simulink library "carnotUIBK_bus"  (R2023b)
settings: Solver=VariableStepAuto  StartTime=0.0  StopTime=10.0  RelTol=1e-3  EnableMultiTasking=on
values from neighbouring files (symbols this model uses):
  A = 7*10*2    (= 140)    [theta_ground_v1.m]    (also in xlswrite1.m = num2cell(data))
  amb_factor = 1    [DOOR.m]    (also in WALL.m; WINDOW.m = 0)
  area = obj.width * obj.height    [DOOR.m]    (also in RES.m = []; ROOM.m = 0; THERMALZONE.m = area + room(kk).area; WALL.m = area - obj.doors(jj).calc_area())
  B = A/(0.5 * P)    (= 8.23529411765)    [theta_ground_v1.m]
  boundary = BOUNDARY()    [BUILDING.m]    (also in WALL.m = '')
  building = obj    [BUILDING.m]    (also in create_building_automatic.m = building.save(); ini_building_automatic.m = building.add_variant_hvac(building.variant_hvac, hvac); load_building_automatic.m = building.save())
  C = zeros(1,length(d)+1)    [CONSTRUCTION.m]    (also in DOOR.m = [0 0 0]; WALL.m = [0 0 0]; WINDOW.m = [0 0 0])
  control = 2    [GAIN.m]    (also in GAINS.m)
  cp = str2num(value)    [CONSTRUCTION.m]
  height = 0    [DOOR.m]    (also in ROOM.m; THERMALZONE.m; WALL.m; WINDOW.m)
  p = [timevec_weather weather(:,12)]    [BOUNDARY.m]    (also in WEATHER.m = 0; init_carnotUIBK.m = cell2mat(carnotUIBKpaths(i,2)))
  rho = str2num(value)    [CONSTRUCTION.m]    (also in theta_ground_v1.m = 2000)
  type = 1    [CONSTRUCTION.m]    (also in GAINS.m = raw_moisture{ii,3}; STRUCTURE.m = 0)
  view_factor = 1    [DOOR.m]    (also in WINDOW.m = 0)
  wall = []    [ROOM.m]
  z = obj.Z    [WALL.m]    (also in theta_ground_v1.m = 0)
  zone = obj.zone(ind)    [THERMALZONE.m]
undefined symbols (not defined in the file or in its folder): const, Dd, get_building, mdot_air, mdot_CO2, mdot_H2O, mdot_VOC, pos, Qdot_C, Qdot_H, Qdot_I_electricity, Qdot_I_light, Qdot_I_person, Qdot_S, Qdot_T_ground, Qdot_T_internal, Qdot_T_neighbour, Qdot_T_opaque, Qdot_T_window, Qdot_V_infiltration, Qdot_V_mech, Qdot_V_window, Qdotc, Qdotr, r_frame, solar_ratio, solar_ratio1, solar_ratio2, Tc, Tr, Ts, Uvalue, wallsurface, window, window_height, window_heigth, window_width, windowsurface, x_CO2, x_H2O, x_VOC
libraries: $bdroot x134, carnot x87, simulink_extras x14, slpidlib x4, simulink x3
(part 10 of 12)

== system carnotUIBK_bus/wall_zone/hygrothermal model/alpha_i/alpha_i_horizontal ==
  note: (W/m^2)
  note: Convective and radiative heat transfer at the INDOOR SURFACE of a VERTICAL OUTER WALL
  note: CONVENTION:
      | Qdot > 0 and qdots < 0, if Ts > T (heat flows from wall surface to room node),
      | Qdot < 0 and qdots > 0, if Ts < T (heat flows from room node to wall surface).
  note: s: surface
      | c: convective
      | r: radiative
  note: dynamic, convective heat transfer coefficients according to: Glück B.: Wärmeübergangskoeffizienten an thermisch aktiven Bauteiloberflächen
      | und der Übergang zu Basiskennlinien für die Wärmestromdichte; gi Gesundheits-Ingenieur; 128. Jahrgang 2007, Heft 1, Seiten 1-10
  Ts : Inport
  AIB : Inport  Port=2
  Qdot sol : Inport  Port=3
  phis : Inport  Port=4
  1/wallsurface : Gain  Gain=1/wallsurface  SaturateOnIntegerOverflow=on  OutDataTypeStr=Inherit: Same as input  ParamDataTypeStr=Inherit: Same as input
  Add : Sum  Commented=on  Inputs=+-
  Bus Assignment2 : BusAssignment  AssignedSignals=Qdotc,Qdotr,mdot_H2O
  Bus Selector : BusSelector  OutputSignals=Tc,Tr,p,x_H2O
  Fcn : Fcn  Expr=1.6*(abs(u(1)-u(2)))^0.3
  Fcn1 : Fcn  Expr=(273.15+u(1))^4-(273.15+u(2))^4
  Gain2 : Gain  Commented=on  Gain=0.01
  Mux2 : Mux  Inputs=2
  Mux3 : Mux  Inputs=2
  Product : Product  InputSameDT=on  RndMeth=Zero  SaturateOnIntegerOverflow=on  OutDataTypeStr=Inherit: Same as first input
  Product1 : Product  InputSameDT=on  RndMeth=Zero  SaturateOnIntegerOverflow=on  OutDataTypeStr=Inherit: Same as first input
  Product2 : Product  Commented=on  RndMeth=Zero
  Product3 : Product  Commented=on  RndMeth=Zero
  Product4 : Product  Commented=on  InputSameDT=on  RndMeth=Zero  SaturateOnIntegerOverflow=on  OutDataTypeStr=Inherit: Same as first input
  S_initialize : $bdroot/general/S_initialize  SystemSampleTime=-1  VariantActivationTime=update diagram  AllowFlexibleInterface=on  Latency=0  AutoFrameSizeCalculation=off
  Sum : Sum  Inputs=+-  InputSameDT=on  SaturateOnIntegerOverflow=on  OutDataTypeStr=Inherit: Same as first input
  Sum2 : Sum  Inputs=+--  InputSameDT=on  SaturateOnIntegerOverflow=on  OutDataTypeStr=Inherit: Same as first input
  Switch : Switch  Commented=on  Criteria=u2 > Threshold  SaturateOnIntegerOverflow=off  InputSameDT=off
  emission_in : Gain  Gain=emission_in  SaturateOnIntegerOverflow=on  OutDataTypeStr=Inherit: Same as input  ParamDataTypeStr=Inherit: Same as input
  lewis : Gain  Commented=on  Gain=0.000000007  SaturateOnIntegerOverflow=on  OutDataTypeStr=Inherit: Same as input  ParamDataTypeStr=Inherit: Same as input
  nomassflow : Constant  Value=0
  ps_l : Fcn  Commented=on  Expr=610.0*exp(17.08*(u)/(234.2+(u)))
  ps_s_l : Fcn  Commented=on  Expr=610.0*exp(17.08*(u)/(234.2+(u)))
  sigma : Constant  Value=5.67e-8
  view_factor : Gain  Gain=view_factor  SaturateOnIntegerOverflow=on  OutDataTypeStr=Inherit: Same as input  ParamDataTypeStr=Inherit: Same as input
  wallsurface1 : Gain  Commented=on  Gain=wallsurface  SaturateOnIntegerOverflow=on  OutDataTypeStr=Inherit: Same as input  ParamDataTypeStr=Inherit: Same as input
  wallsurface2 : Gain  Gain=wallsurface  SaturateOnIntegerOverflow=on  OutDataTypeStr=Inherit: Same as input  ParamDataTypeStr=Inherit: Same as input
  wallsurface3 : Gain  Gain=wallsurface  SaturateOnIntegerOverflow=on  OutDataTypeStr=Inherit: Same as input  ParamDataTypeStr=Inherit: Same as input
  x2RelHum_UIBK : carnot/Basic/Material_Properties/x2RelHum  Commented=on
      settings: SourceProductName=Carnot
  qdots : Outport  InitialOutput=0  VectorParamsAs1DForOutWhenUnconnected=off
  "[S]" : Outport  Port=2  InitialOutput=0  VectorParamsAs1DForOutWhenUnconnected=off
  alpha_c : Outport  Port=3  InitialOutput=0  VectorParamsAs1DForOutWhenUnconnected=off
  phi_i_1/100 : Outport  Port=4  InitialOutput=0  VectorParamsAs1DForOutWhenUnconnected=off
  wires:
  wallsurface1/1 -> Switch/1
  view_factor/1 -> Product/1
  phis/1 -> Product3/1, Switch/2
  Product2/1 -> Add/2
  Product3/1 -> Add/1
  ps_s_l/1 -> Product3/2
  ps_l/1 -> Product2/2
  lewis/1 -> wallsurface1/1
  Gain2/1 -> Product2/1, phi_i_1/100/1
  Bus Selector/4 -> x2RelHum_UIBK/3  "<x_H2O>"
  Bus Selector/3 -> x2RelHum_UIBK/2  "<p>"
  x2RelHum_UIBK/1 -> Gain2/1
  Fcn1/1 -> Product/2
  Mux3/1 -> Fcn1/1
  sigma/1 -> emission_in/1
  Sum2/1 -> qdots/1
  AIB/1 -> Bus Selector/1
  Bus Selector/1 -> Sum/2, Mux2/2, x2RelHum_UIBK/1, ps_l/1  "<Tc>"
  emission_in/1 -> view_factor/1
  Product/1 -> wallsurface3/1, Sum2/3  "qdotr"
  Ts/1 -> Sum/1, ps_s_l/1, Mux3/1, Mux2/1  "Ts"
  Sum/1 -> Product1/1  "dTc"
  Bus Selector/2 -> Mux3/2  "<Tr>"
  Mux2/1 -> Fcn/1
  Product1/1 -> wallsurface2/1, Sum2/2  "qdotc"
  Fcn/1 -> alpha_c/1, Product4/1, Product1/2  "hc"
  Qdot sol/1 -> 1/wallsurface/1
  1/wallsurface/1 -> Sum2/1
  Product4/1 -> lewis/1
  Add/1 -> Product4/2
  nomassflow/1 -> Bus Assignment2/4, Switch/3
  S_initialize/1 -> Bus Assignment2/1
  wallsurface2/1 -> Bus Assignment2/2  "Qdotc"
  wallsurface3/1 -> Bus Assignment2/3  "Qdotr"
  Bus Assignment2/1 -> "[S]"/1

== system carnotUIBK_bus/wall_zone/hygrothermal model/alpha_i/alpha_i_up ==
  note: (W/m^2)
  note: Convective and radiative heat transfer at the INDOOR SURFACE of a ceiling
  note: CONVENTION:
      | Qdot > 0 and qdots < 0, if Ts > T (heat flows from wall surface to room node),
      | Qdot < 0 and qdots > 0, if Ts < T (heat flows from room node to wall surface).
  note: s: surface
      | c: convective
      | r: radiative
  note: dynamic, convective heat transfer coefficients according to: Glück B.: Wärmeübergangskoeffizienten an thermisch aktiven Bauteiloberflächen
      | und der Übergang zu Basiskennlinien für die Wärmestromdichte; gi Gesundheits-Ingenieur; 128. Jahrgang 2007, Heft 1, Seiten 1-10
  Ts : Inport
  AIB : Inport  Port=2
  Qdot sol : Inport  Port=3
  phis : Inport  Port=4
  1/wallsurface : Gain  Gain=1/wallsurface  SaturateOnIntegerOverflow=on  OutDataTypeStr=Inherit: Same as input  ParamDataTypeStr=Inherit: Same as input
  Add : Sum  Commented=on  Inputs=+-
  Bus Assignment2 : BusAssignment  AssignedSignals=Qdotc,Qdotr,mdot_H2O
  Bus Selector : BusSelector  OutputSignals=Tc,Tr,p,x_H2O
  Fcn1 : Fcn  Expr=(273.15+u(1))^4-(273.15+u(2))^4
  Gain2 : Gain  Commented=on  Gain=0.01
  Mux2 : Mux  Inputs=2
  Mux3 : Mux  Inputs=2
  Product : Product  InputSameDT=on  RndMeth=Zero  SaturateOnIntegerOverflow=on  OutDataTypeStr=Inherit: Same as first input
  Product1 : Product  InputSameDT=on  RndMeth=Zero  SaturateOnIntegerOverflow=on  OutDataTypeStr=Inherit: Same as first input
  Product2 : Product  Commented=on  RndMeth=Zero
  Product3 : Product  Commented=on  RndMeth=Zero
  Product4 : Product  Commented=on  InputSameDT=on  RndMeth=Zero  SaturateOnIntegerOverflow=on  OutDataTypeStr=Inherit: Same as first input
  S_initialize : $bdroot/general/S_initialize  SystemSampleTime=-1  VariantActivationTime=update diagram  AllowFlexibleInterface=on  Latency=0  AutoFrameSizeCalculation=off
  Sum : Sum  Inputs=+-  InputSameDT=on  SaturateOnIntegerOverflow=on  OutDataTypeStr=Inherit: Same as first input
  Sum2 : Sum  Inputs=+--  InputSameDT=on  SaturateOnIntegerOverflow=on  OutDataTypeStr=Inherit: Same as first input
  Switch : Switch  Commented=on  Criteria=u2 > Threshold  SaturateOnIntegerOverflow=off  InputSameDT=off
  Switch1 : Switch  SaturateOnIntegerOverflow=off  InputSameDT=off
  emission_in : Gain  Gain=emission_in  SaturateOnIntegerOverflow=on  OutDataTypeStr=Inherit: Same as input  ParamDataTypeStr=Inherit: Same as input
  heat flux downwards : Fcn  Expr=0.54*(abs(u(1)-u(2))^0.31)
  heat flux upwards : Fcn  Expr=2*(abs(u(1)-u(2))^0.31)
  lewis : Gain  Commented=on  Gain=0.000000007  SaturateOnIntegerOverflow=on  OutDataTypeStr=Inherit: Same as input  ParamDataTypeStr=Inherit: Same as input
  nomassflow : Constant  Value=0
  ps_l : Fcn  Commented=on  Expr=610.0*exp(17.08*(u)/(234.2+(u)))
  ps_s_l : Fcn  Commented=on  Expr=610.0*exp(17.08*(u)/(234.2+(u)))
  sigma : Constant  Value=5.67e-8
  view_factor : Gain  Gain=view_factor  SaturateOnIntegerOverflow=on  OutDataTypeStr=Inherit: Same as input  ParamDataTypeStr=Inherit: Same as input
  wallsurface1 : Gain  Commented=on  Gain=wallsurface  SaturateOnIntegerOverflow=on  OutDataTypeStr=Inherit: Same as input  ParamDataTypeStr=Inherit: Same as input
  wallsurface2 : Gain  Gain=wallsurface  SaturateOnIntegerOverflow=on  OutDataTypeStr=Inherit: Same as input  ParamDataTypeStr=Inherit: Same as input
  wallsurface3 : Gain  Gain=wallsurface  SaturateOnIntegerOverflow=on  OutDataTypeStr=Inherit: Same as input  ParamDataTypeStr=Inherit: Same as input
  x2RelHum_UIBK : carnot/Basic/Material_Properties/x2RelHum  Commented=on
      settings: SourceProductName=Carnot
  qdots : Outport  InitialOutput=0  VectorParamsAs1DForOutWhenUnconnected=off
  "[S]" : Outport  Port=2  InitialOutput=0  VectorParamsAs1DForOutWhenUnconnected=off
  alpha_c : Outport  Port=3  InitialOutput=0  VectorParamsAs1DForOutWhenUnconnected=off
  phi_i_1/100 : Outport  Port=4  InitialOutput=0  VectorParamsAs1DForOutWhenUnconnected=off
  wires:
  wallsurface1/1 -> Switch/1
  view_factor/1 -> Product/1
  phis/1 -> Product3/1, Switch/2
  Product2/1 -> Add/2
  Product3/1 -> Add/1
  ps_s_l/1 -> Product3/2
  ps_l/1 -> Product2/2
  lewis/1 -> wallsurface1/1
  Gain2/1 -> Product2/1, phi_i_1/100/1
  Bus Selector/4 -> x2RelHum_UIBK/3  "<x_H2O>"
  Bus Selector/3 -> x2RelHum_UIBK/2  "<p>"
  x2RelHum_UIBK/1 -> Gain2/1
  Fcn1/1 -> Product/2
  Mux3/1 -> Fcn1/1
  sigma/1 -> emission_in/1
  Sum2/1 -> qdots/1
  AIB/1 -> Bus Selector/1
  Bus Selector/1 -> Sum/2, Mux2/2, x2RelHum_UIBK/1, ps_l/1  "<Tc>"
  emission_in/1 -> view_factor/1
  Ts/1 -> Sum/1, ps_s_l/1, Mux3/1, Mux2/1  "Ts"
  Bus Selector/2 -> Mux3/2  "<Tr>"
  Mux2/1 -> heat flux downwards/1, heat flux upwards/1
  Switch1/1 -> Product1/2, Product4/1, alpha_c/1  "hc"
  Qdot sol/1 -> 1/wallsurface/1
  1/wallsurface/1 -> Sum2/1
  Sum/1 -> Switch1/2, Product1/1  "dTc"
  heat flux upwards/1 -> Switch1/3
  heat flux downwards/1 -> Switch1/1
  Product4/1 -> lewis/1
  Add/1 -> Product4/2
  S_initialize/1 -> Bus Assignment2/1
  Product/1 -> Sum2/3, wallsurface3/1  "qdotr"
  wallsurface3/1 -> Bus Assignment2/3  "Qdotr"
  wallsurface2/1 -> Bus Assignment2/2  "Qdotc"
  Product1/1 -> wallsurface2/1, Sum2/2  "qdotc"
  nomassflow/1 -> Bus Assignment2/4, Switch/3
  Bus Assignment2/1 -> "[S]"/1

== system carnotUIBK_bus/window/window_CARNOT/alfa_window_in/Irradiation into room ==
  note: Solar radiation into zone
  "[I_t]" : Inport
  "[tau]" : Inport  Port=2
  Demux : Demux  Outputs=3
      settings: DisplayOption=none
  Demux1 : Demux  Outputs=2
      settings: DisplayOption=none
  Product5 : Product  InputSameDT=on  SaturateOnIntegerOverflow=on  OutDataTypeStr=Inherit: Same as first input
  Product6 : Product  InputSameDT=on  SaturateOnIntegerOverflow=on  OutDataTypeStr=Inherit: Same as first input
  Sum1 : Sum  InputSameDT=on  SaturateOnIntegerOverflow=on  OutDataTypeStr=Inherit: Same as first input
  gvalue of glass : Gain  Gain=gvalue  SaturateOnIntegerOverflow=on  OutDataTypeStr=Inherit: Same as input  ParamDataTypeStr=Inherit: Same as input
  tau,dir(0) : Terminator
  qdot_sol : Outport  InitialOutput=0  VectorParamsAs1DForOutWhenUnconnected=off
  wires:
  gvalue of glass/1 -> qdot_sol/1
  Sum1/1 -> gvalue of glass/1
  "[tau]"/1 -> Demux/1
  Demux/1 -> Product5/1  "tau_dir(teta)"
  Demux/2 -> tau,dir(0)/1
  "[I_t]"/1 -> Demux1/1
  Demux1/2 -> Product6/1  "Idfu_t"
  Demux1/1 -> Product5/2  "Idir_t"
  Demux/3 -> Product6/2  "tau_dfu"
  Product6/1 -> Sum1/2
  Product5/1 -> Sum1/1

== system carnotUIBK_bus/window/window_CARNOT/alfa_window_in/transmission coefficient 1-2-3-4-layer(s) ==
  teta : Inport
  LUT_taualfa : Subsystem  mask(LOOK UP TABLE){}
      mask help:
      | This block delivers the standardized LIGHT TRANSMISSION COEFFICIENT of a window glass with 1, 2, 3 or 4 layers depending on the incidence angle. Each layer may be 3 to 8 mm thick.
      |
      | teta:    incidence angle = angle between surface normal and
      |                 incidence, degree
      | numlayer: number of layers within the window glass, [1,4].
      | tau:    transmission of glass layer stack, [0,1]
  Mux : Mux  Inputs=3
  numlayer : Constant  Value=numlayer
  perpendicular : Constant  Value=0
  tau,dfu - angle : Constant  Value=60
  "[tau]" : Outport  InitialOutput=0  VectorParamsAs1DForOutWhenUnconnected=off
  wires:
  LUT_taualfa/1(tau) -> "[tau]"/1
  numlayer/1 -> LUT_taualfa/2(numlayer)
  Mux/1 -> LUT_taualfa/1(teta)
  perpendicular/1 -> Mux/2
  tau,dfu - angle/1 -> Mux/3
  teta/1 -> Mux/1

== system carnotUIBK_bus/window/window_CARNOT/alfa_window_out/qp rad ==
  Ta : Inport
  Tw : Inport  Port=2
  Tsky : Inport  Port=3
  Sum : Sum  Inputs=-++  InputSameDT=on  SaturateOnIntegerOverflow=on  OutDataTypeStr=Inherit: Same as first input
  Ta*f : Fcn  Expr=(amb_factor)*(273.15+u[1])^4
  Tsky*f : Fcn  Expr=(1-amb_factor)*(273.15+u[1])^4
  Tw kel : Fcn  Expr=(273.15+u[1])^4
  qdot : Fcn  Expr=u(1)*emission_out*5.67e-8
  qprad : Outport  InitialOutput=0  VectorParamsAs1DForOutWhenUnconnected=off
  wires:
  Tsky/1 -> Tsky*f/1
  Ta/1 -> Ta*f/1
  qdot/1 -> qprad/1
  Sum/1 -> qdot/1
  Ta*f/1 -> Sum/3
  Tw/1 -> Tw kel/1
  Tw kel/1 -> Sum/1
  Tsky*f/1 -> Sum/2

== system carnotUIBK_bus/window/window_TF/alfa_window_in/transmission_absorption ==
  note: Assumption:
      | 1. gvalue = gvalue(0)
      | 2. gvalue(teta) / gvalue = tau(teta) / tau(0)
  note: 1. solar radiation into room (behind window glass layers)
      | 2. absorbed solar radiation flowing from inner window surface into zone
  sun_t : Inport
  WDB : Inport  Port=2
  control : Inport  Port=3
  Demux : Demux  Outputs=2
      settings: DisplayOption=none
  Demux1 : Demux  Outputs=3
      settings: DisplayOption=none
  LUT_taualfa : Subsystem  mask(LOOK UP TABLE){}
      mask help:
      | Normalized RADIATION TRANSMISSION COEFFICIENT of a window glass layer stack with 1, 2, 3 or 4 layers depending on the incidence angle.
      |
      | teta		: incidence angle = angle between surface normal and
      | 	                incidence direction, degree
      | numlayer	: number of layers within the window glass, [1,4].
      | tau		: transmission of glass layer stack, [0,1]
      |
      | NOTE: This block is defined for pane thickness between 3 and 6 mm.
  Mux : Mux  Inputs=2
  Product{1..4,7..8} (6 alike) : Product  InputSameDT=on  RndMeth=Zero  SaturateOnIntegerOverflow=on  OutDataTypeStr=Inherit: Same as first input
  Product11 : Product  Inputs=**  InputSameDT=on  RndMeth=Zero  SaturateOnIntegerOverflow=on  OutDataTypeStr=Inherit: Same as first input
  Shading : Subsystem
  Sum : Sum  Inputs=+-  InputSameDT=on  SaturateOnIntegerOverflow=on  OutDataTypeStr=Inherit: Same as first input
  Sum3 : Sum  InputSameDT=on  SaturateOnIntegerOverflow=on  OutDataTypeStr=Inherit: Same as first input
  const1 : Constant  Value=gvalue
  numlayer : Constant  Value=numpanes
  tau(0) : Gain  Gain=tauzero  SaturateOnIntegerOverflow=on  OutDataTypeStr=Inherit: Same as input  ParamDataTypeStr=Inherit: Same as input
  teta(taudfu) : Constant  Value=60
  qdot_abs : Outport  VectorParamsAs1DForOutWhenUnconnected=off
  qdot_sol : Outport  Port=2  VectorParamsAs1DForOutWhenUnconnected=off
  wires:
  control/1 -> Shading/2(control)
  WDB/1 -> Shading/1(WDB)
  Shading/3(f_g) -> Product4/2
  const1/1 -> Product4/1
  Product4/1 -> Product11/1
  Shading/4(f_tau) -> Product3/2
  Shading/2(f_dfu) -> Product1/2
  Shading/1(f_dir) -> Product2/2
  Product2/1 -> Product7/2
  Demux1/2 -> Product2/1  "Idir_t"
  Product1/1 -> Product8/2
  Demux1/3 -> Product1/1  "Idfu_t"
  Product3/1 -> qdot_sol/1, Sum/2
  tau(0)/1 -> Product3/1
  sun_t/1 -> Demux1/1
  LUT_taualfa/1(tau_norm) -> Demux/1  "Qdot_sol"
  Demux/1 -> Product7/1  "tau_norm(teta)"
  Product7/1 -> Sum3/1
  Product8/1 -> Sum3/2
  Sum3/1 -> Product11/2, tau(0)/1
  Demux/2 -> Product8/1  "tau_norm(60)"
  Product11/1 -> Sum/1  "qdot_room"
  Sum/1 -> qdot_abs/1
  Demux1/1 -> Mux/1  "teta"
  teta(taudfu)/1 -> Mux/2
  numlayer/1 -> LUT_taualfa/1(numlpanes)
  Mux/1 -> LUT_taualfa/2(teta)

== system carnotUIBK_bus/window/window_TF/alfa_window_out/qp rad ==
  Ta : Inport
  Tw : Inport  Port=2
  Tsky : Inport  Port=3
  Sum : Sum  Inputs=-++  InputSameDT=on  SaturateOnIntegerOverflow=on  OutDataTypeStr=Inherit: Same as first input
  Ta*f : Fcn  Expr=(amb_factor)*(273.15+u[1])^4
  Tsky*f : Fcn  Expr=(1-amb_factor)*(273.15+u[1])^4
  Tw kel : Fcn  Expr=(273.15+u[1])^4
  qdot : Fcn  Expr=u(1)*emission_out*5.67e-8
  qprad : Outport  InitialOutput=0  VectorParamsAs1DForOutWhenUnconnected=off
  wires:
  Tsky/1 -> Tsky*f/1
  Ta/1 -> Ta*f/1
  qdot/1 -> qprad/1
  Sum/1 -> qdot/1
  Ta*f/1 -> Sum/3
  Tw/1 -> Tw kel/1
  Tw kel/1 -> Sum/1
  Tsky*f/1 -> Sum/2

== system carnotUIBK_bus/window/window_TF_shading/alfa_window_in/transmission_absorption ==
  note: Assumption:
      | 1. gvalue = gvalue(0)
      | 2. gvalue(teta) / gvalue = tau(teta) / tau(0)
  note: 1. solar radiation into room (behind window glass layers)
      | 2. absorbed solar radiation flowing from inner window surface into zone
  sun_t : Inport
  WDB : Inport  Port=2
  control : Inport  Port=3
  Demux : Demux  Outputs=2
      settings: DisplayOption=none
  Demux1 : Demux  Outputs=3
      settings: DisplayOption=none
  LUT_taualfa : Subsystem  mask(LOOK UP TABLE){}
      mask help:
      | Normalized RADIATION TRANSMISSION COEFFICIENT of a window glass layer stack with 1, 2, 3 or 4 layers depending on the incidence angle.
      |
      | teta		: incidence angle = angle between surface normal and
      | 	                incidence direction, degree
      | numlayer	: number of layers within the window glass, [1,4].
      | tau		: transmission of glass layer stack, [0,1]
      |
      | NOTE: This block is defined for pane thickness between 3 and 6 mm.
  Mux : Mux  Inputs=2
  Product{1..4,7..8} (6 alike) : Product  InputSameDT=on  RndMeth=Zero  SaturateOnIntegerOverflow=on  OutDataTypeStr=Inherit: Same as first input
  Product11 : Product  Inputs=**  InputSameDT=on  RndMeth=Zero  SaturateOnIntegerOverflow=on  OutDataTypeStr=Inherit: Same as first input
  Shading : Subsystem
  Sum : Sum  Inputs=+-  InputSameDT=on  SaturateOnIntegerOverflow=on  OutDataTypeStr=Inherit: Same as first input
  Sum3 : Sum  InputSameDT=on  SaturateOnIntegerOverflow=on  OutDataTypeStr=Inherit: Same as first input
  const1 : Constant  Value=gvalue
  numlayer : Constant  Value=numpanes
  tau(0) : Gain  Gain=tauzero  SaturateOnIntegerOverflow=on  OutDataTypeStr=Inherit: Same as input  ParamDataTypeStr=Inherit: Same as input
  teta(taudfu) : Constant  Value=60
  qdot_abs : Outport  VectorParamsAs1DForOutWhenUnconnected=off
  qdot_sol : Outport  Port=2  VectorParamsAs1DForOutWhenUnconnected=off
  wires:
  control/1 -> Shading/2(control)
  WDB/1 -> Shading/1(WDB)
  Shading/3(f_g) -> Product4/2
  const1/1 -> Product4/1
  Product4/1 -> Product11/1
  Shading/4(f_tau) -> Product3/2
  Shading/2(f_dfu) -> Product1/2
  Shading/1(f_dir) -> Product2/2
  Product2/1 -> Product7/2
  Demux1/2 -> Product2/1  "Idir_t"
  Product1/1 -> Product8/2
  Demux1/3 -> Product1/1  "Idfu_t"
  Product3/1 -> qdot_sol/1, Sum/2
  tau(0)/1 -> Product3/1
  sun_t/1 -> Demux1/1
  LUT_taualfa/1(tau_norm) -> Demux/1  "Qdot_sol"
  Demux/1 -> Product7/1  "tau_norm(teta)"
  Product7/1 -> Sum3/1
  Product8/1 -> Sum3/2
  Sum3/1 -> Product11/2, tau(0)/1
  Demux/2 -> Product8/1  "tau_norm(60)"
  Product11/1 -> Sum/1  "qdot_room"
  Sum/1 -> qdot_abs/1
  Demux1/1 -> Mux/1  "teta"
  teta(taudfu)/1 -> Mux/2
  numlayer/1 -> LUT_taualfa/1(numlpanes)
  Mux/1 -> LUT_taualfa/2(teta)

== system carnotUIBK_bus/window/window_TF_shading/alfa_window_out/qp rad ==
  Ta : Inport
  Tw : Inport  Port=2
  Tsky : Inport  Port=3
  Sum : Sum  Inputs=-++  InputSameDT=on  SaturateOnIntegerOverflow=on  OutDataTypeStr=Inherit: Same as first input
  Ta*f : Fcn  Expr=(amb_factor)*(273.15+u[1])^4
  Tsky*f : Fcn  Expr=(1-amb_factor)*(273.15+u[1])^4
  Tw kel : Fcn  Expr=(273.15+u[1])^4
  qdot : Fcn  Expr=u(1)*emission_out*5.67e-8
  qprad : Outport  InitialOutput=0  VectorParamsAs1DForOutWhenUnconnected=off
  wires:
  Tsky/1 -> Tsky*f/1
  Ta/1 -> Ta*f/1
  qdot/1 -> qprad/1
  Sum/1 -> qdot/1
  Ta*f/1 -> Sum/3
  Tw/1 -> Tw kel/1
  Tw kel/1 -> Sum/1
  Tsky*f/1 -> Sum/2

== system carnotUIBK_bus/gain/People/W//ppl (activity)/LUT_Qdot_dry/Look-Up Table Qdot_dry ==
  Rows : Inport
  Cols : Inport  Port=2
  Look-Up Table (2-D) : Lookup2D  RowIndex=x  ColumnIndex=y  Table=t
  U : Outport  VectorParamsAs1DForOutWhenUnconnected=off
  wires:
  Look-Up Table (2-D)/1 -> U/1
  Cols/1 -> Look-Up Table (2-D)/2
  Rows/1 -> Look-Up Table (2-D)/1

== system carnotUIBK_bus/gain/People/W//ppl (activity)/LUT_Qdot_hum1/Look-Up Table Qdot_hum ==
  Rows : Inport
  Cols : Inport  Port=2
  Look-Up Table (2-D) : Lookup2D  RowIndex=x  ColumnIndex=y  Table=t
  U : Outport  VectorParamsAs1DForOutWhenUnconnected=off
  wires:
  Rows/1 -> Look-Up Table (2-D)/1
  Cols/1 -> Look-Up Table (2-D)/2
  Look-Up Table (2-D)/1 -> U/1

== system carnotUIBK_bus/gain/People/W//ppl (activity)/LUT_mdot_H2O/Look-Up Table mdot_H2O ==
  Rows : Inport
  Cols : Inport  Port=2
  Look-Up Table (2-D) : Lookup2D  RowIndex=x  ColumnIndex=y  Table=t
  U : Outport  VectorParamsAs1DForOutWhenUnconnected=off
  wires:
  Rows/1 -> Look-Up Table (2-D)/1
  Cols/1 -> Look-Up Table (2-D)/2
  Look-Up Table (2-D)/1 -> U/1

== system carnotUIBK_bus/gain/People/W//ppl (constant)/LUT_mdot_H2O/Look-Up Table mdot_H2O ==
  Rows : Inport
  Cols : Inport  Port=2
  Look-Up Table (2-D) : Lookup2D  RowIndex=x  ColumnIndex=y  Table=t
  U : Outport  VectorParamsAs1DForOutWhenUnconnected=off
  wires:
  Rows/1 -> Look-Up Table (2-D)/1
  Cols/1 -> Look-Up Table (2-D)/2
  Look-Up Table (2-D)/1 -> U/1

== system carnotUIBK_bus/infiltration/infiltration_pressure/infiltration_pressure/dP_infiltration/calculate wind_coeff ==
  wind_angle : Inport
  additional_coeff_wind : Inport  Port=2
  facade_angle : Inport  Port=3
  Cin (see ASHRAE 24.4) : Constant  Value=0.2
  Cs (see ASHRAE 24.5) : Polyval  Coefs=[0.0000005, -0.00008, -0.0074, 0.674]
  Product2 : Product
  Subtract : Sum  Inputs=-++
  Subtract1 : Sum  Inputs=+-
  const_angle : Constant  Value=180
  wind_coeff : Outport  VectorParamsAs1DForOutWhenUnconnected=off
  wires:
  wind_angle/1 -> Subtract/1
  additional_coeff_wind/1 -> Product2/2
  Product2/1 -> wind_coeff/1
  facade_angle/1 -> Subtract/3
  Subtract/1 -> Cs (see ASHRAE 24.5)/1
  const_angle/1 -> Subtract/2
  Cin (see ASHRAE 24.4)/1 -> Subtract1/2
  Subtract1/1 -> Product2/1
  Cs (see ASHRAE 24.5)/1 -> Subtract1/1

== system carnotUIBK_bus/wall_zone/R-C model/alpha_e/alpha_e_AMBIENT/qp rad ==
  Ta : Inport
  Tw : Inport  Port=2
  Tsky : Inport  Port=3
  Sum : Sum  Inputs=-++  InputSameDT=on  SaturateOnIntegerOverflow=on  OutDataTypeStr=Inherit: Same as first input
  Ta*f : Fcn  Expr=(amb_factor)*(273.15+u[1])^4
  Tsky*f : Fcn  Expr=(1-amb_factor)*(273.15+u[1])^4
  Tw kel : Fcn  Expr=(273.15+u[1])^4
  qdot : Fcn  Expr=u(1)*emission_out*5.67e-8
  qprad : Outport  InitialOutput=0  VectorParamsAs1DForOutWhenUnconnected=off
  wires:
  Tsky*f/1 -> Sum/2
  Tw kel/1 -> Sum/1
  Tw/1 -> Tw kel/1
  Ta*f/1 -> Sum/3
  Sum/1 -> qdot/1
  qdot/1 -> qprad/1
  Ta/1 -> Ta*f/1
  Tsky/1 -> Tsky*f/1

== system carnotUIBK_bus/wall_zone/R-C model/alpha_e/alpha_e_AMBIENT/wall_surfrad ==
  note: (3 = Sky model
      | Perez)
  note: Direct and diffuse
      | radiation on a
      | tilted and shaded
      | outdoor surface
  WDB : Inport
  Bus Selector : BusSelector  OutputSignals=Solar_Radiation_direct_surface,Solar_Radiation_diffuse_surface  OutputAsBus=on
  Radiation_on_Inclined_Surface : carnot/Weather/Radiation_on_Inclined_Surface  sky=Perez 1990  reflect=0.2
      settings: SourceProductName=Carnot
  Sum : Sum  Inputs=1  InputSameDT=on  SaturateOnIntegerOverflow=on  OutDataTypeStr=Inherit: Same as first input
  position : Constant  Value=pos
  Idir,t+Idfu,t : Outport  InitialOutput=0  VectorParamsAs1DForOutWhenUnconnected=off
  wires:
  Bus Selector/1 -> Sum/1
  Radiation_on_Inclined_Surface/1 -> Bus Selector/1
  Sum/1 -> Idir,t+Idfu,t/1
  WDB/1 -> Radiation_on_Inclined_Surface/1
  position/1 -> Radiation_on_Inclined_Surface/2

== system carnotUIBK_bus/wall_zone/R-C model/alpha_e/alpha_e_INTERNAL/alpha_i ==
  Ts : Inport
  AIB : Inport  Port=2
  Qdot sol : Inport  Port=3
  phis : Inport  Port=4
  alpha_i_down : Subsystem  VariantControl=V_zXXX_wXXX_hti2  mask(ALFA){}
      mask help:
      | Convective and radiative heat transfer at the INDOOR SURFACE of a VERTICAL OUTER WALL.
      |
      | [AIV] : conditions of zone node,
      | Ts : temperature of wall surface, °C,
      | qdots : specific heat flow into wall construction, W/m^2,
      | [S] : heat and air flow to zone node.
  alpha_i_horizontal : Subsystem  VariantControl=V_zXXX_wXXX_hti0  mask(ALFA){}
      mask help:
      | Convective and radiative heat transfer at the INDOOR SURFACE of a VERTICAL OUTER WALL.
      |
      | [AIV] : conditions of zone node,
      | Ts : temperature of wall surface, °C,
      | qdots : specific heat flow into wall construction, W/m^2,
      | [S] : heat and air flow to zone node.
  alpha_i_up : Subsystem  VariantControl=V_zXXX_wXXX_hti1  mask(ALFA){}
      mask help:
      | Convective and radiative heat transfer at the INDOOR SURFACE of a VERTICAL OUTER WALL.
      |
      | [AIV] : conditions of zone node,
      | Ts : temperature of wall surface, °C,
      | qdots : specific heat flow into wall construction, W/m^2,
      | [S] : heat and air flow to zone node.
  qdots : Outport  VectorParamsAs1DForOutWhenUnconnected=off
  "[S]" : Outport  Port=2  VectorParamsAs1DForOutWhenUnconnected=off
  alpha_c : Outport  Port=3  VectorParamsAs1DForOutWhenUnconnected=off
  phi_i_1/100 : Outport  Port=4  VectorParamsAs1DForOutWhenUnconnected=off

== system carnotUIBK_bus/wall_zone/R-C model/alpha_e/alpha_e_NEIGHBOUR/alpha_i ==
  Ts : Inport
  AIB : Inport  Port=2
  Qdot sol : Inport  Port=3
  phis : Inport  Port=4
  alpha_i_down : Subsystem  VariantControl=V_zXXX_wXXX_hti2  mask(ALFA){}
      mask help:
      | Convective and radiative heat transfer at the INDOOR SURFACE of a VERTICAL OUTER WALL.
      |
      | [AIV] : conditions of zone node,
      | Ts : temperature of wall surface, °C,
      | qdots : specific heat flow into wall construction, W/m^2,
      | [S] : heat and air flow to zone node.
  alpha_i_horizontal : Subsystem  VariantControl=V_zXXX_wXXX_hti0  mask(ALFA){}
      mask help:
      | Convective and radiative heat transfer at the INDOOR SURFACE of a VERTICAL OUTER WALL.
      |
      | [AIV] : conditions of zone node,
      | Ts : temperature of wall surface, °C,
      | qdots : specific heat flow into wall construction, W/m^2,
      | [S] : heat and air flow to zone node.
  alpha_i_up : Subsystem  VariantControl=V_zXXX_wXXX_hti1  mask(ALFA){}
      mask help:
      | Convective and radiative heat transfer at the INDOOR SURFACE of a VERTICAL OUTER WALL.
      |
      | [AIV] : conditions of zone node,
      | Ts : temperature of wall surface, °C,
      | qdots : specific heat flow into wall construction, W/m^2,
      | [S] : heat and air flow to zone node.
  qdots : Outport  VectorParamsAs1DForOutWhenUnconnected=off
  "[S]" : Outport  Port=2  VectorParamsAs1DForOutWhenUnconnected=off
  alpha_c : Outport  Port=3  VectorParamsAs1DForOutWhenUnconnected=off
  phi_i_1/100 : Outport  Port=4  VectorParamsAs1DForOutWhenUnconnected=off

== system carnotUIBK_bus/wall_zone/hygrothermal model/alpha_e/alpha_e_AMBIENT/qp rad ==
  Ta : Inport
  Tw : Inport  Port=2
  Tsky : Inport  Port=3
  Sum : Sum  Inputs=-++  InputSameDT=on  SaturateOnIntegerOverflow=on  OutDataTypeStr=Inherit: Same as first input
  Ta*f : Fcn  Expr=(amb_factor)*(273.15+u[1])^4
  Tsky*f : Fcn  Expr=(1-amb_factor)*(273.15+u[1])^4
  Tw kel : Fcn  Expr=(273.15+u[1])^4
  qdot : Fcn  Expr=u(1)*emission_out*5.67e-8
  qprad : Outport  InitialOutput=0  VectorParamsAs1DForOutWhenUnconnected=off
  wires:
  Tsky*f/1 -> Sum/2
  Tw kel/1 -> Sum/1
  Tw/1 -> Tw kel/1
  Ta*f/1 -> Sum/3
  Sum/1 -> qdot/1
  qdot/1 -> qprad/1
  Ta/1 -> Ta*f/1
  Tsky/1 -> Tsky*f/1

== system carnotUIBK_bus/wall_zone/hygrothermal model/alpha_e/alpha_e_AMBIENT/wall_surfrad ==
  note: (3 = Sky model
      | Perez)
  note: Direct and diffuse
      | radiation on a
      | tilted and shaded
      | outdoor surface
  WDB : Inport
  Bus Selector : BusSelector  OutputSignals=Solar_Radiation_direct_surface,Solar_Radiation_diffuse_surface  OutputAsBus=on
  Radiation_on_Inclined_Surface : carnot/Weather/Radiation_on_Inclined_Surface  sky=Perez 1990  reflect=0.2
      settings: SourceProductName=Carnot
  Sum : Sum  Inputs=1  InputSameDT=on  SaturateOnIntegerOverflow=on  OutDataTypeStr=Inherit: Same as first input
  position : Constant  Value=pos
  Idir,t+Idfu,t : Outport  InitialOutput=0  VectorParamsAs1DForOutWhenUnconnected=off
  wires:
  Bus Selector/1 -> Sum/1
  Radiation_on_Inclined_Surface/1 -> Bus Selector/1
  Sum/1 -> Idir,t+Idfu,t/1
  WDB/1 -> Radiation_on_Inclined_Surface/1
  position/1 -> Radiation_on_Inclined_Surface/2

== system carnotUIBK_bus/wall_zone/hygrothermal model/alpha_e/alpha_e_INTERNAL/alpha_i ==
  Ts : Inport
  AIB : Inport  Port=2
  Qdot sol : Inport  Port=3
  phis : Inport  Port=4
  alpha_i_down : Subsystem  VariantControl=V_zXXX_wXXX_hti2  mask(ALFA){}
      mask help:
      | Convective and radiative heat transfer at the INDOOR SURFACE of a VERTICAL OUTER WALL.
      |
      | [AIV] : conditions of zone node,
      | Ts : temperature of wall surface, °C,
      | qdots : specific heat flow into wall construction, W/m^2,
      | [S] : heat and air flow to zone node.
  alpha_i_horizontal : Subsystem  VariantControl=V_zXXX_wXXX_hti0  mask(ALFA){}
      mask help:
      | Convective and radiative heat transfer at the INDOOR SURFACE of a VERTICAL OUTER WALL.
      |
      | [AIV] : conditions of zone node,
      | Ts : temperature of wall surface, °C,
      | qdots : specific heat flow into wall construction, W/m^2,
      | [S] : heat and air flow to zone node.
  alpha_i_up : Subsystem  VariantControl=V_zXXX_wXXX_hti1  mask(ALFA){}
      mask help:
      | Convective and radiative heat transfer at the INDOOR SURFACE of a VERTICAL OUTER WALL.
      |
      | [AIV] : conditions of zone node,
      | Ts : temperature of wall surface, °C,
      | qdots : specific heat flow into wall construction, W/m^2,
      | [S] : heat and air flow to zone node.
  qdots : Outport  VectorParamsAs1DForOutWhenUnconnected=off
  "[S]" : Outport  Port=2  VectorParamsAs1DForOutWhenUnconnected=off
  alpha_c : Outport  Port=3  VectorParamsAs1DForOutWhenUnconnected=off
  phi_i_1/100 : Outport  Port=4  VectorParamsAs1DForOutWhenUnconnected=off

== system carnotUIBK_bus/wall_zone/hygrothermal model/alpha_e/alpha_e_NEIGHBOUR/alpha_i ==
  Ts : Inport
  AIB : Inport  Port=2
  Qdot sol : Inport  Port=3
  phis : Inport  Port=4
  alpha_i_down : Subsystem  VariantControl=V_zXXX_wXXX_hti2  mask(ALFA){}
      mask help:
      | Convective and radiative heat transfer at the INDOOR SURFACE of a VERTICAL OUTER WALL.
      |
      | [AIV] : conditions of zone node,
      | Ts : temperature of wall surface, °C,
      | qdots : specific heat flow into wall construction, W/m^2,
      | [S] : heat and air flow to zone node.
  alpha_i_horizontal : Subsystem  VariantControl=V_zXXX_wXXX_hti0  mask(ALFA){}
      mask help:
      | Convective and radiative heat transfer at the INDOOR SURFACE of a VERTICAL OUTER WALL.
      |
      | [AIV] : conditions of zone node,
      | Ts : temperature of wall surface, °C,
      | qdots : specific heat flow into wall construction, W/m^2,
      | [S] : heat and air flow to zone node.
  alpha_i_up : Subsystem  VariantControl=V_zXXX_wXXX_hti1  mask(ALFA){}
      mask help:
      | Convective and radiative heat transfer at the INDOOR SURFACE of a VERTICAL OUTER WALL.
      |
      | [AIV] : conditions of zone node,
      | Ts : temperature of wall surface, °C,
      | qdots : specific heat flow into wall construction, W/m^2,
      | [S] : heat and air flow to zone node.
  qdots : Outport  VectorParamsAs1DForOutWhenUnconnected=off
  "[S]" : Outport  Port=2  VectorParamsAs1DForOutWhenUnconnected=off
  alpha_c : Outport  Port=3  VectorParamsAs1DForOutWhenUnconnected=off
  phi_i_1/100 : Outport  Port=4  VectorParamsAs1DForOutWhenUnconnected=off

== system carnotUIBK_bus/window/window_CARNOT/alfa_window_in/transmission coefficient 1-2-3-4-layer(s)/LUT_taualfa ==
  note: NOTE: The TAUALFA-Lookup-table is calculated with "taualfa.m"
      | for 4 mm glass, but you can use it also for  3, 4, 6 or 8 mm glass.
      | The mistake is neglectable (see results in "taulut.m").
  note: transmission coefficient TAUALFA of a window glass with 1,2,3 or 4 layers
  note: (from: Duffie / Beckman: Solar Engineering of Thermal Processes, 1991
  teta : Inport
  numlayer : Inport  Port=2
  "TAUALFA 1-2-3-4 layers, standardized to 1.0, (4 mm float glass, no dirt absorption, 97% room absorption)" : Subsystem  mask(Lookup Table (2-D)){x=[0:10:90], y=[1:4], t=[1.0000 1.0000 1.0000 1.0000; 0.9996 0.9991 0.9987 0.9983; 0.9979 0.9961 0.9945 0.9929; 0.9937 0.9894 0.9861 0.9836; 0.9839 0.9753 0.9704 0.9680; 0.9608 0.9438 0.9365 0.9361; 0.9061 0.8679 0.8484 0.8413; 0.7755 0.6821 0.6182 0.5717; 0.4807 0.3277 0.2324 0.1688; 0 0 0 0]}
      mask prompts: x "Row:"; y "Column:"; t "Table:"
      mask help: Performs 2-D linear interpolation of input values using the specified input/output table. Extrapolation is performed outside the table boundaries.
      mask init:
      | [r,c]=size(t);
      | xt=reshape(x,prod(size(x)),1);
      | xi=xt(:,ones(1,c));
      | minx=min(x); maxx=max(x);
      | mint=min(min(t)); maxt=max(max(t));
      mask Display: plot(xi,t,[minx maxx],[mint mint],[minx minx],[mint maxt])
  tau : Outport  InitialOutput=0  VectorParamsAs1DForOutWhenUnconnected=off
  wires:
  teta/1 -> "TAUALFA 1-2-3-4 layers, standardized to 1.0, (4 mm float glass, no dirt absorption, 97% room absorption)"/1(Rows)
  numlayer/1 -> "TAUALFA 1-2-3-4 layers, standardized to 1.0, (4 mm float glass, no dirt absorption, 97% room absorption)"/2(Cols)
  "TAUALFA 1-2-3-4 layers, standardized to 1.0, (4 mm float glass, no dirt absorption, 97% room absorption)"/1(Out1) -> tau/1

== system carnotUIBK_bus/window/window_TF/alfa_window_in/transmission_absorption/LUT_taualfa ==
  note: NOTE:
      | TAUALFA-Lookup-table calculated with "taualfa.m":
      |   a) 4mm float glass (error neglectable if glass thickness is 3 or 6mm),
      |   b) no dirt absorption on glass surfaces,
      |   c) 100% room absorption,
      |   d) normalized to tau(0).
      |
      | From: Duffie / Beckman: Solar Engineering of Thermal Processes, 1991
  note: Normalized radiation transmission TAUALFA
      | of a window glass stack with 1,2,3 or 4 layers
  numlpanes : Inport
  teta : Inport  Port=2
  TAUALFA 1-2-3-4 layers : Lookup2D  RowIndex=[0:10:90]  ColumnIndex=[1:4]  Table="[1  1  1  1;.99955 .99912  .9987 .99827;.99787  .9961 .99449 .99298;.99364 .98941 .98618 .98366;.98364 .97519 .97041 .96824;.9601 .94337 .93638 .93624;.90423 .86634 .84734 .84064;.77129 .67843 .61507 .56891;.47436  .3235 .22952 .16682;0  0  0  0]"
  tau_norm : Outport  VectorParamsAs1DForOutWhenUnconnected=off
  wires:
  teta/1 -> TAUALFA 1-2-3-4 layers/1
  numlpanes/1 -> TAUALFA 1-2-3-4 layers/2
  TAUALFA 1-2-3-4 layers/1 -> tau_norm/1

== system carnotUIBK_bus/window/window_TF/alfa_window_in/transmission_absorption/Shading ==
  WDB : Inport
  control : Inport  Port=2
  Bus Selector : BusSelector  OutputSignals=Zenith_Angle
  Demux : Demux
  Mux : Mux  Inputs=2
  S-Function : S-Function  FunctionName=venetian  Parameters=bli_a, bli_b, bli_c, bli_d, bli_alpha, bli_refl, shad_type, type_glazing, tau_shad  SFunctionDeploymentMode=off  EnableBusSupport=off
  f_dir : Outport  VectorParamsAs1DForOutWhenUnconnected=off
  f_dfu : Outport  Port=2  VectorParamsAs1DForOutWhenUnconnected=off
  f_g : Outport  Port=3  VectorParamsAs1DForOutWhenUnconnected=off
  f_tau : Outport  Port=4  VectorParamsAs1DForOutWhenUnconnected=off
  wires:
  WDB/1 -> Bus Selector/1
  Bus Selector/1 -> Mux/2  "<Zenith_Angle>"
  control/1 -> Mux/1
  Mux/1 -> S-Function/1
  S-Function/1 -> Demux/1
  Demux/1 -> f_dir/1
  Demux/2 -> f_dfu/1
  Demux/3 -> f_g/1
  Demux/4 -> f_tau/1

== system carnotUIBK_bus/window/window_TF_shading/alfa_window_in/transmission_absorption/LUT_taualfa ==
  note: NOTE:
      | TAUALFA-Lookup-table calculated with "taualfa.m":
      |   a) 4mm float glass (error neglectable if glass thickness is 3 or 6mm),
      |   b) no dirt absorption on glass surfaces,
      |   c) 100% room absorption,
      |   d) normalized to tau(0).
      |
      | From: Duffie / Beckman: Solar Engineering of Thermal Processes, 1991
  note: Normalized radiation transmission TAUALFA
      | of a window glass stack with 1,2,3 or 4 layers
  numlpanes : Inport
  teta : Inport  Port=2
  TAUALFA 1-2-3-4 layers : Lookup2D  RowIndex=[0:10:90]  ColumnIndex=[1:4]  Table="[1  1  1  1;.99955 .99912  .9987 .99827;.99787  .9961 .99449 .99298;.99364 .98941 .98618 .98366;.98364 .97519 .97041 .96824;.9601 .94337 .93638 .93624;.90423 .86634 .84734 .84064;.77129 .67843 .61507 .56891;.47436  .3235 .22952 .16682;0  0  0  0]"
  tau_norm : Outport  VectorParamsAs1DForOutWhenUnconnected=off
  wires:
  teta/1 -> TAUALFA 1-2-3-4 layers/1
  numlpanes/1 -> TAUALFA 1-2-3-4 layers/2
  TAUALFA 1-2-3-4 layers/1 -> tau_norm/1

== system carnotUIBK_bus/window/window_TF_shading/alfa_window_in/transmission_absorption/Shading ==
  WDB : Inport
  control : Inport  Port=2
  Bus Selector : BusSelector  OutputSignals=Zenith_Angle
  Demux : Demux
  Mux : Mux  Inputs=2
  S-Function : S-Function  FunctionName=venetian  Parameters=bli_a, bli_b, bli_c, bli_d, bli_alpha, bli_refl, shad_type, type_glazing, tau_shad  SFunctionDeploymentMode=off  EnableBusSupport=off
  f_dir : Outport  VectorParamsAs1DForOutWhenUnconnected=off
  f_dfu : Outport  Port=2  VectorParamsAs1DForOutWhenUnconnected=off
  f_g : Outport  Port=3  VectorParamsAs1DForOutWhenUnconnected=off
  f_tau : Outport  Port=4  VectorParamsAs1DForOutWhenUnconnected=off
  wires:
  WDB/1 -> Bus Selector/1
  Bus Selector/1 -> Mux/2  "<Zenith_Angle>"
  control/1 -> Mux/1
  Mux/1 -> S-Function/1
  S-Function/1 -> Demux/1
  Demux/1 -> f_dir/1
  Demux/2 -> f_dfu/1
  Demux/3 -> f_g/1
  Demux/4 -> f_tau/1

== system carnotUIBK_bus/wall_zone/R-C model/alpha_e/alpha_e_INTERNAL/alpha_i/alpha_i_down ==
  note: (W/m^2)
  note: Convective and radiative heat transfer at the INDOOR SURFACE of a VERTICAL OUTER WALL
  note: CONVENTION:
      | Qdot > 0 and qdots < 0, if Ts > T (heat flows from wall surface to room node),
      | Qdot < 0 and qdots > 0, if Ts < T (heat flows from room node to wall surface).
  note: s: surface
      | c: convective
      | r: radiative
  note: dynamic, convective heat transfer coefficients according to: Glück B.: Wärmeübergangskoeffizienten an thermisch aktiven Bauteiloberflächen
      | und der Übergang zu Basiskennlinien für die Wärmestromdichte; gi Gesundheits-Ingenieur; 128. Jahrgang 2007, Heft 1, Seiten 1-10
  Ts : Inport
  AIB : Inport  Port=2
  Qdot sol : Inport  Port=3
  phis : Inport  Port=4
  1/wallsurface : Gain  Gain=1/wallsurface  SaturateOnIntegerOverflow=on  OutDataTypeStr=Inherit: Same as input  ParamDataTypeStr=Inherit: Same as input
  Add : Sum  Commented=on  Inputs=+-
  Bus Assignment2 : BusAssignment  AssignedSignals=Qdotc,Qdotr,Qdot_T_internal,mdot_H2O
  Bus Selector : BusSelector  OutputSignals=Tc,Tr,p,x_H2O
  Fcn1 : Fcn  Expr=(273.15+u(1))^4-(273.15+u(2))^4
  Gain2 : Gain  Commented=on  Gain=0.01
  Mux2 : Mux  Inputs=2
  Mux3 : Mux  Inputs=2
  Product : Product  InputSameDT=on  RndMeth=Zero  SaturateOnIntegerOverflow=on  OutDataTypeStr=Inherit: Same as first input
  Product1 : Product  InputSameDT=on  RndMeth=Zero  SaturateOnIntegerOverflow=on  OutDataTypeStr=Inherit: Same as first input
  Product2 : Product  Commented=on  RndMeth=Zero
  Product3 : Product  Commented=on  RndMeth=Zero
  S_initialize : $bdroot/general/S_initialize  SystemSampleTime=-1  VariantActivationTime=update diagram  AllowFlexibleInterface=on  Latency=0  AutoFrameSizeCalculation=off
  Sum : Sum  Inputs=+-  InputSameDT=on  SaturateOnIntegerOverflow=on  OutDataTypeStr=Inherit: Same as first input
  Sum2 : Sum  Inputs=+--  InputSameDT=on  SaturateOnIntegerOverflow=on  OutDataTypeStr=Inherit: Same as first input
  Switch : Switch  Commented=on  Criteria=u2 > Threshold  SaturateOnIntegerOverflow=off  InputSameDT=off
  Switch1 : Switch  SaturateOnIntegerOverflow=off  InputSameDT=off
  Wallsurf : Gain  Gain=wallsurface  SaturateOnIntegerOverflow=on  OutDataTypeStr=Inherit: Same as input  ParamDataTypeStr=Inherit: Same as input
  emission_in : Gain  Gain=emission_in  SaturateOnIntegerOverflow=on  OutDataTypeStr=Inherit: Same as input  ParamDataTypeStr=Inherit: Same as input
  heat flux downwards : Fcn  Expr=0.54*(abs(u(1)-u(2))^0.31)
  heat flux upwards : Fcn  Expr=2*(abs(u(1)-u(2))^0.31)
  lewis : Gain  Commented=on  Gain=0.000000007  SaturateOnIntegerOverflow=on  OutDataTypeStr=Inherit: Same as input  ParamDataTypeStr=Inherit: Same as input
  nomassflow : Constant  Value=0
  ps_l : Fcn  Commented=on  Expr=610.0*exp(17.08*(u)/(234.2+(u)))
  ps_s_l : Fcn  Commented=on  Expr=610.0*exp(17.08*(u)/(234.2+(u)))
  sigma : Constant  Value=5.67e-8
  view_factor : Gain  Gain=view_factor  SaturateOnIntegerOverflow=on  OutDataTypeStr=Inherit: Same as input  ParamDataTypeStr=Inherit: Same as input
  wallsurface : Gain  Gain=wallsurface  SaturateOnIntegerOverflow=on  OutDataTypeStr=Inherit: Same as input  ParamDataTypeStr=Inherit: Same as input
  wallsurface1 : Gain  Commented=on  Gain=wallsurface  SaturateOnIntegerOverflow=on  OutDataTypeStr=Inherit: Same as input  ParamDataTypeStr=Inherit: Same as input
  wallsurface2 : Gain  Gain=wallsurface  SaturateOnIntegerOverflow=on  OutDataTypeStr=Inherit: Same as input  ParamDataTypeStr=Inherit: Same as input
  x2RelHum_UIBK : carnot/Basic/Material_Properties/x2RelHum  Commented=on
      settings: SourceProductName=Carnot
  qdots : Outport  InitialOutput=0  VectorParamsAs1DForOutWhenUnconnected=off
  "[S]" : Outport  Port=2  InitialOutput=0  VectorParamsAs1DForOutWhenUnconnected=off
  alpha_c : Outport  Port=3  InitialOutput=0  VectorParamsAs1DForOutWhenUnconnected=off
  phi_i_1/100 : Outport  Port=4  InitialOutput=0  VectorParamsAs1DForOutWhenUnconnected=off
  wires:
  wallsurface1/1 -> Switch/1
  view_factor/1 -> Product/1
  phis/1 -> Product3/1, Switch/2
  Add/1 -> lewis/1
  Product2/1 -> Add/2
  Product3/1 -> Add/1
  ps_s_l/1 -> Product3/2
  ps_l/1 -> Product2/2
  lewis/1 -> wallsurface1/1
  Gain2/1 -> Product2/1, phi_i_1/100/1
  Bus Selector/4 -> x2RelHum_UIBK/3  "<x_H2O>"
  Bus Selector/3 -> x2RelHum_UIBK/2  "<p>"
  x2RelHum_UIBK/1 -> Gain2/1
  Fcn1/1 -> Product/2
  Mux3/1 -> Fcn1/1
  sigma/1 -> emission_in/1
  AIB/1 -> Bus Selector/1
  Bus Selector/1 -> Sum/2, Mux2/2, x2RelHum_UIBK/1, ps_l/1  "<Tc>"
  emission_in/1 -> view_factor/1
  Product/1 -> wallsurface/1, Sum2/3  "qdotr"
  Ts/1 -> Sum/1, ps_s_l/1, Mux3/1, Mux2/1  "Ts"
  Bus Selector/2 -> Mux3/2  "<Tr>"
  Mux2/1 -> heat flux downwards/1, heat flux upwards/1
  Switch1/1 -> Product1/2, alpha_c/1  "hc"
  Qdot sol/1 -> 1/wallsurface/1
  1/wallsurface/1 -> Sum2/1
  Sum/1 -> Switch1/2, Product1/1  "dTc"
  heat flux upwards/1 -> Switch1/1
  heat flux downwards/1 -> Switch1/3
  Product1/1 -> wallsurface2/1, Sum2/2  "Qdotc"
  Bus Assignment2/1 -> "[S]"/1
  Sum2/1 -> Wallsurf/1, qdots/1
  nomassflow/1 -> Bus Assignment2/5, Switch/3
  wallsurface2/1 -> Bus Assignment2/2
  S_initialize/1 -> Bus Assignment2/1
  wallsurface/1 -> Bus Assignment2/3  "Qdotr]"
  Wallsurf/1 -> Bus Assignment2/4  "Qdotint]"
